simulink model "rlinvpend"  (R2019b)
settings: Solver=VariableStepAuto  StartTime=0.0  StopTime=Tf  RelTol=1e-3
model workspace (MATLAB code in the model file):
  | mCart = 1;
  | mPend = 1;
  | g = 9.81;
  | L = 0.5;
  | theta0 = 180;
  | Kd = 10;
values from neighbouring files (symbols this model uses):
  alpha_a = 0.002    [invertedpndlm_MrAsadmfile.m]
  alpha_c = 0.001    [invertedpndlm_MrAsadmfile.m]
  epsilon = 0.001    [invertedpndlm_MrAsadmfile.m]
  m = 0.1    [invertedpndlm_MrAsadmfile.m]
  s = tf('s')    [invertedpndlm_MrAsadmfile.m]
  Ts = 0.02    [invertedpndlm_MrAsadmfile.m]
undefined symbols (not defined in the file or in its folder): X, Y, Z
libraries: sm_lib x11, nesl_utility x7, fuzblock x3, rllib x2, simulink x2
settings Model: Creator=ndoshi  LastModifiedBy=hp
settings DataIOCC: TimeSaveName=T  SignalLoggingName=LoggedSigs
settings DebuggingCC: ArithmeticOperatorsInVariantConditions=warning
settings SFSimCC: CustomCodeUndefinedFunction=UseInterfaceOnly

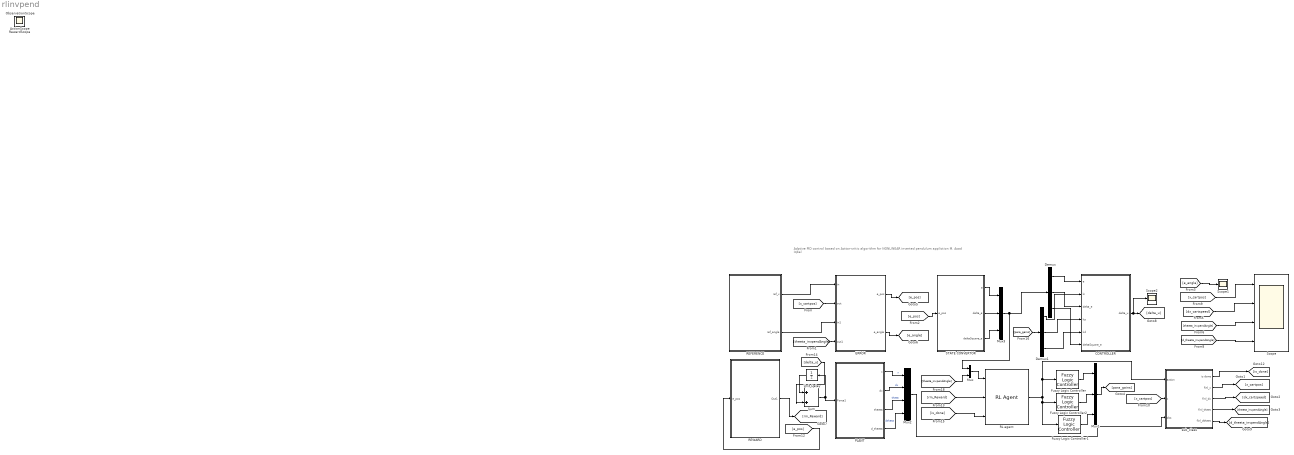
== system rlinvpend ==
  note: Adptive PID control based on Acttor-critic algorithm for NONLINEAR inverted pendulum appliction
      | M. Asad Iqbal
  CONTROLLER : Subsystem
  Demux : Demux  Outputs=3
  Demux1 : Demux  Outputs=3
  ERROR : Subsystem
  Fuzzy Logic Controller : fuzblock/Fuzzy Logic  Controller  FIS=p_n  OutputSampleNumber=101  DataType=double  FuzzifiedInputs=off  RuleFiringStrengths=off  RuleOutputs=off  AggregatedOutputs=off  SimulateUsing=Interpreted execution  OutOfRangeInputValueMessage=warning  NoRuleFiredMessage=warning  EmptyOutputFuzzySetMessage=warning
  Fuzzy Logic Controller1 : fuzblock/Fuzzy Logic  Controller  FIS=d_n  OutputSampleNumber=101  DataType=double  FuzzifiedInputs=off  RuleFiringStrengths=off  RuleOutputs=off  AggregatedOutputs=off  SimulateUsing=Interpreted execution  OutOfRangeInputValueMessage=warning  NoRuleFiredMessage=warning  EmptyOutputFuzzySetMessage=warning
  Fuzzy Logic Controller2 : fuzblock/Fuzzy Logic  Controller  FIS=i_ni  OutputSampleNumber=101  DataType=double  FuzzifiedInputs=off  RuleFiringStrengths=off  RuleOutputs=off  AggregatedOutputs=off  SimulateUsing=Interpreted execution  OutOfRangeInputValueMessage=warning  NoRuleFiredMessage=warning  EmptyOutputFuzzySetMessage=warning
  Mux : Mux  Inputs=2
  Mux1 : Mux  Inputs=3
  Mux2 : Mux
  Mux3 : Mux  Inputs=3
  PLANT : Subsystem
  REFERENCE : Subsystem
  REWARD : Subsystem
  "RL agent " : rllib/RL Agent  Agent=agent  ProvideReward=on  ProvideIsDone=on  ProvideCumRwd=off  TreatAsDirectFeedthrough=on  CollectLoggedSignals=on  CollectModelStates=on
      settings: SourceProductName=The database C:\Users\ddavis\AppData\Roaming\MathWorks\MATLAB\R2018b\slblocks_master.db is locked, or a table in the database is locked. (database is locked)
  STATE CONVERTOR : Subsystem
  Scope : Scope  NumInputPorts=4
  Scope1 : Scope
  Scope2 : Scope
  Sum : Sum  Inputs=|++
  Unit Delay : UnitDelay  SampleTime=-1  HasFrameUpgradeWarning=on
  sub_class : Subsystem
  ActionScope : Scope
  ObservationScope : Scope
  RewardScope : Scope
  wires:
  PLANT/1(x) -> Mux2/1  "x"
  PLANT/4(d_theeta) -> Mux2/4  "dtheta"
  [para_gains] -> Demux1/1
  STATE CONVERTOR/3(deltaSquare_e) -> Mux3/3
  [theeta_invpendAngle] -> ERROR/4(out1)
  Demux/3 -> CONTROLLER/6(deltaSquare_e)
  Demux/1 -> CONTROLLER/1("e ")
  [e_pos] -> REWARD/1(e_pos)
  [d_theeta_invpendAngle] -> Scope/4
  [dx_cartspeed] -> Scope/2
  Demux1/3 -> CONTROLLER/5(kd)
  Unit Delay/1 -> Sum/1
  [theeta_invpendAngle] -> Scope/3
  [x_cartpos] -> Scope/1
  CONTROLLER/1(delta_u) -> Scope2/1, [delta_u]
  Demux1/2 -> CONTROLLER/4(kp)
  Sum/1 -> Unit Delay/1, PLANT/1(Force1)
  [delta_u] -> Sum/2
  Demux/2 -> CONTROLLER/3(delta_e)
  [x_cartpos] -> ERROR/2(out)
  REFERENCE/2(ref_angle) -> ERROR/3(in1)
  STATE CONVERTOR/2(delta_e) -> Mux3/2
  [e_pos] -> STATE CONVERTOR/1("e_pos ")
  ERROR/1(e_pos) -> [e_pos]
  ERROR/2(e_angle) -> [e_angle]
  REFERENCE/1(ref_x) -> ERROR/1(in)
  REWARD/1(Out1) -> [rm_Reward]
  Demux1/1 -> CONTROLLER/2(ki)
  PLANT/2(dx) -> Mux2/2  "dx"
  STATE CONVERTOR/1(e) -> Mux3/1
  PLANT/3(theeta) -> Mux2/3  "theta"
  [theeta_invpendAngle] -> Mux/2
  sub_class/1(is done) -> [is_done]
  sub_class/2(finl_x) -> [x_cartpos]
  sub_class/3(finl_dx) -> [dx_cartspeed]
  Mux/1 -> "RL agent "/1
  [rm_Reward] -> "RL agent "/2
  Mux3/1 -> Mux/1, Demux/1
  [is_done] -> "RL agent "/3
  sub_class/4(finl_theet) -> [theeta_invpendAngle]
  [x_cartpos] -> sub_class/2(x)
  sub_class/5(finl_dtheet) -> [d_theeta_invpendAngle]
  Mux2/1 -> sub_class/3(obs)
  "RL agent "/1 -> sub_class/1("action "), Fuzzy Logic Controller/1, Fuzzy Logic Controller1/1, Fuzzy Logic Controller2/1
  Fuzzy Logic Controller/1 -> Mux1/1
  Fuzzy Logic Controller2/1 -> Mux1/2
  Fuzzy Logic Controller1/1 -> Mux1/3
  [e_angle] -> Scope1/1
  Mux1/1 -> [para_gains]

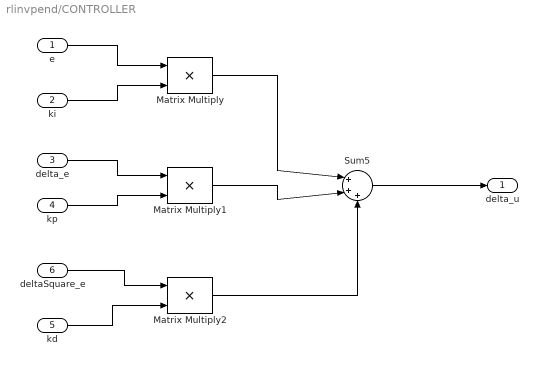
== system rlinvpend/CONTROLLER ==
  "e " : Inport
  ki : Inport  Port=2
  delta_e : Inport  Port=3
  kp : Inport  Port=4
  kd : Inport  Port=5
  deltaSquare_e : Inport  Port=6
  Matrix Multiply : Product
  Matrix Multiply1 : Product
  Matrix Multiply2 : Product
  Sum5 : Sum  Inputs=|+++
  delta_u : Outport
  wires:
  Sum5/1 -> delta_u/1
  deltaSquare_e/1 -> Matrix Multiply2/1
  delta_e/1 -> Matrix Multiply1/1
  "e "/1 -> Matrix Multiply/1
  ki/1 -> Matrix Multiply/2
  kd/1 -> Matrix Multiply2/2
  Matrix Multiply/1 -> Sum5/1
  kp/1 -> Matrix Multiply1/2
  Matrix Multiply1/1 -> Sum5/2
  Matrix Multiply2/1 -> Sum5/3

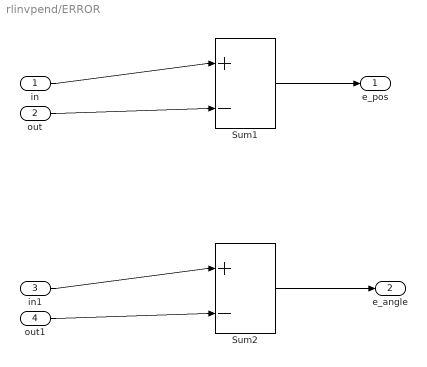
== system rlinvpend/ERROR ==
  in : Inport
  out : Inport  Port=2
  in1 : Inport  Port=3
  out1 : Inport  Port=4
  Sum1 : Sum  Inputs=|+-
  Sum2 : Sum  Inputs=|+-
  e_pos : Outport
  e_angle : Outport  Port=2
  wires:
  in/1 -> Sum1/1
  out/1 -> Sum1/2
  in1/1 -> Sum2/1
  out1/1 -> Sum2/2
  Sum1/1 -> e_pos/1
  Sum2/1 -> e_angle/1

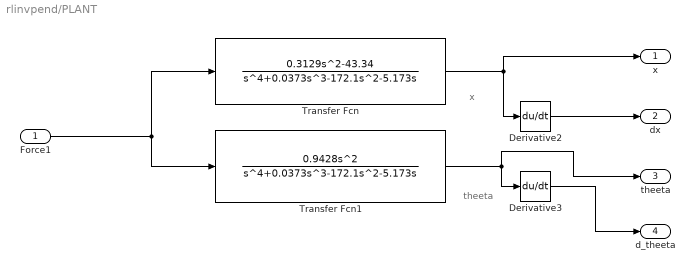
== system rlinvpend/PLANT ==
  note: theeta
  note: x
  Force1 : Inport
  Derivative2 : Derivative
  Derivative3 : Derivative
  Transfer Fcn : TransferFcn  Numerator=[0 0 0.3129 0 -43.34]  Denominator=[1 0.0373 -172.1 -5.173 0]
  Transfer Fcn1 : TransferFcn  Numerator=[0 0 0.9428 0 0]  Denominator=[1 0.0373 -172.1 -5.173 0]
  x : Outport
  dx : Outport  Port=2
  theeta : Outport  Port=3
  d_theeta : Outport  Port=4
  wires:
  Transfer Fcn1/1 -> theeta/1, Derivative3/1
  Transfer Fcn/1 -> x/1, Derivative2/1
  Derivative3/1 -> d_theeta/1
  Derivative2/1 -> dx/1
  Force1/1 -> Transfer Fcn1/1, Transfer Fcn/1

== system rlinvpend/REFERENCE ==
  "Step Input Displacement " : Step  Time=0.005  Before=0.2  After=0  SampleTime=0
  TILT ANGLE : Step  Time=0  After=0  SampleTime=0
  ref_x : Outport
  ref_angle : Outport  Port=2
  wires:
  TILT ANGLE/1 -> ref_angle/1
  "Step Input Displacement "/1 -> ref_x/1

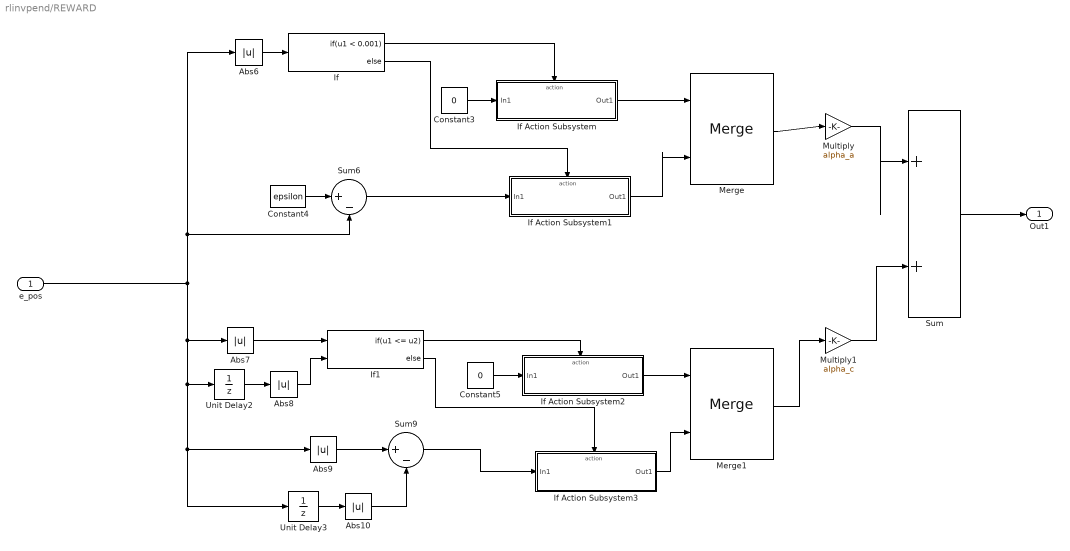
== system rlinvpend/REWARD ==
  e_pos : Inport
  Abs{6..10} (5 alike) : Abs
  Constant3 : Constant  Value=0
  Constant4 : Constant  Value=epsilon
  Constant5 : Constant  Value=0
  If : If  IfExpression=u1 < 0.001
  If Action Subsystem : Subsystem  TreatAsAtomicUnit=on
  If Action Subsystem1 : Subsystem  TreatAsAtomicUnit=on
  If Action Subsystem2 : Subsystem  TreatAsAtomicUnit=on
  If Action Subsystem3 : Subsystem  TreatAsAtomicUnit=on
  If1 : If  NumInputs=2  IfExpression=u1 <= u2
  Merge : Merge
  Merge1 : Merge
  Multiply : Gain  Gain=alpha_a
  Multiply1 : Gain  Gain=alpha_c
  Sum : Sum  Inputs=|++
  Sum6 : Sum  Inputs=|+-
  Sum9 : Sum  Inputs=|+-
  Unit Delay2 : UnitDelay  SampleTime=-1  HasFrameUpgradeWarning=on
  Unit Delay3 : UnitDelay  SampleTime=-1  HasFrameUpgradeWarning=on
  Out1 : Outport
  wires:
  Sum6/1 -> If Action Subsystem1/1(In1)
  If/2 -> If Action Subsystem1/Action
  Constant4/1 -> Sum6/1
  e_pos/1 -> Abs6/1, Sum6/2, Abs9/1, Unit Delay3/1, Unit Delay2/1, Abs7/1
  Unit Delay3/1 -> Abs10/1
  If Action Subsystem/1(Out1) -> Merge/1
  Constant3/1 -> If Action Subsystem/1(In1)
  Multiply1/1 -> Sum/2
  If Action Subsystem3/1(Out1) -> Merge1/2
  Unit Delay2/1 -> Abs8/1
  Sum/1 -> Out1/1
  If/1 -> If Action Subsystem/Action
  If Action Subsystem1/1(Out1) -> Merge/2
  Abs6/1 -> If/1
  Multiply/1 -> Sum/1
  Merge/1 -> Multiply/1
  Merge1/1 -> Multiply1/1
  Sum9/1 -> If Action Subsystem3/1(In1)
  Abs8/1 -> If1/2
  Abs7/1 -> If1/1
  If Action Subsystem2/1(Out1) -> Merge1/1
  Constant5/1 -> If Action Subsystem2/1(In1)
  Abs10/1 -> Sum9/2
  If1/1 -> If Action Subsystem2/Action
  If1/2 -> If Action Subsystem3/Action
  Abs9/1 -> Sum9/1

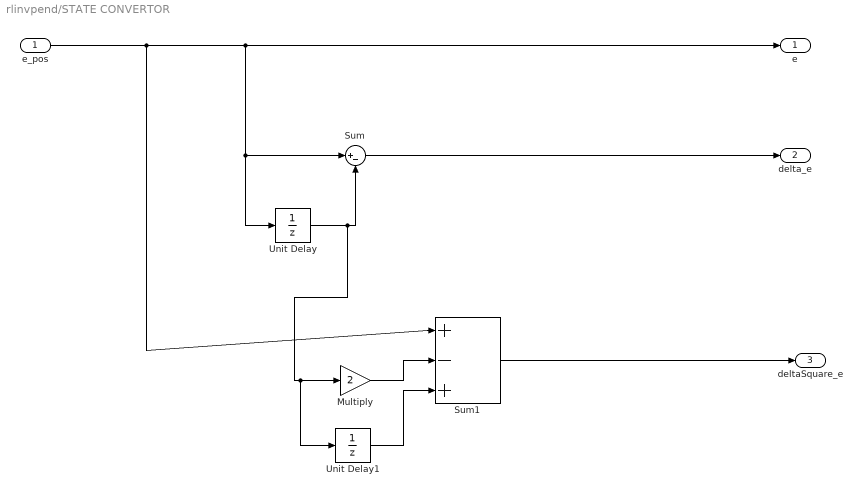
== system rlinvpend/STATE CONVERTOR ==
  "e_pos " : Inport
  Multiply : Gain  Gain=2
  Sum : Sum  Inputs=|+-
  Sum1 : Sum  Inputs=|+-+
  Unit Delay : UnitDelay  SampleTime=-1  HasFrameUpgradeWarning=on
  Unit Delay1 : UnitDelay  SampleTime=-1  HasFrameUpgradeWarning=on
  e : Outport
  delta_e : Outport  Port=2
  deltaSquare_e : Outport  Port=3
  wires:
  "e_pos "/1 -> Sum1/1, Sum/1, Unit Delay/1, e/1
  Unit Delay/1 -> Unit Delay1/1, Multiply/1, Sum/2
  Sum/1 -> delta_e/1
  Sum1/1 -> deltaSquare_e/1
  Multiply/1 -> Sum1/2
  Unit Delay1/1 -> Sum1/3

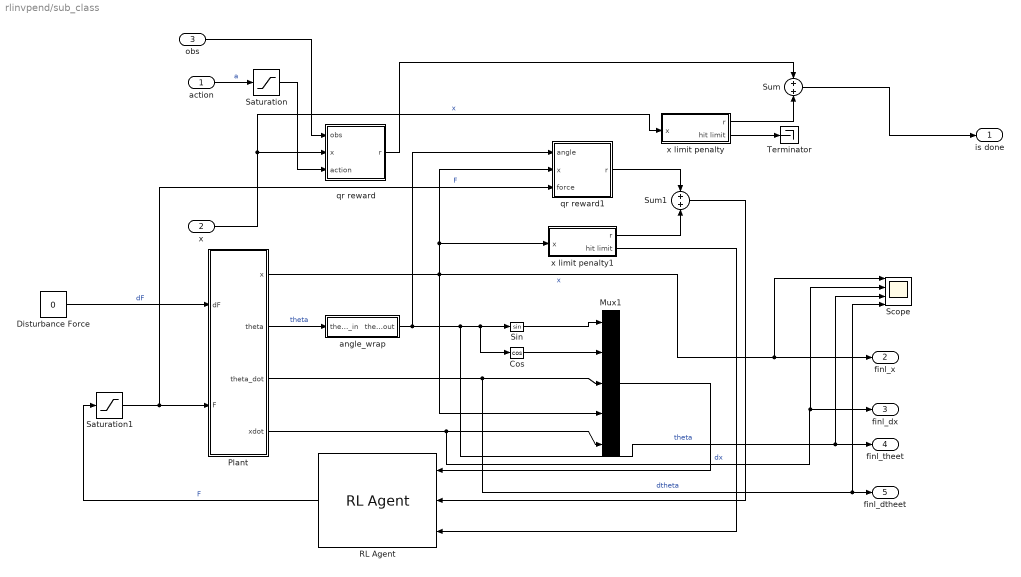
== system rlinvpend/sub_class ==
  "action " : Inport
  x : Inport  Port=2
  obs : Inport  Port=3
  Cos : Trigonometry  Operator=cos
  Disturbance Force : Constant  Value=0
  Mux1 : Mux  Inputs=5
  Plant : Subsystem
  RL Agent : rllib/RL Agent  Agent=agent_dp  ProvideReward=on  ProvideIsDone=on  ProvideCumRwd=off  TreatAsDirectFeedthrough=on  CollectLoggedSignals=on  CollectModelStates=on
      settings: SourceProductName=The database C:\Users\ddavis\AppData\Roaming\MathWorks\MATLAB\R2018b\slblocks_master.db is locked, or a table in the database is locked. (database is locked)
  Saturation : Saturate  UpperLimit=15  LowerLimit=-15
  Saturation1 : Saturate  UpperLimit=15  LowerLimit=-15
  Scope : Scope  NumInputPorts=4
  Sin : Trigonometry
  Sum : Sum
  Sum1 : Sum
  Terminator : Terminator
  angle_wrap : Subsystem
  qr reward : Subsystem
  qr reward1 : Subsystem
  x limit penalty : Subsystem
  x limit penalty1 : Subsystem
  is done : Outport  VectorParamsAs1DForOutWhenUnconnected=off
  finl_x : Outport  Port=2
  finl_dx : Outport  Port=3
  finl_theet : Outport  Port=4
  finl_dtheet : Outport  Port=5
  wires:
  obs/1 -> qr reward/1(obs)
  x/1 -> x limit penalty/1(x), qr reward/2(x)  "x"
  Saturation/1 -> qr reward/3(action)
  "action "/1 -> Saturation/1  "a"
  qr reward/1(r) -> Sum/1
  x limit penalty/1(r) -> Sum/2
  Sum/1 -> is done/1
  x limit penalty1/2(hit limit) -> RL Agent/3
  Sum1/1 -> RL Agent/2
  Mux1/1 -> RL Agent/1
  x limit penalty1/1(r) -> Sum1/2
  qr reward1/1(r) -> Sum1/1
  RL Agent/1 -> Saturation1/1  "F"
  Saturation1/1 -> qr reward1/3(force), Plant/2(F)  "F"
  Cos/1 -> Mux1/2
  Sin/1 -> Mux1/1
  Plant/4(xdot) -> Scope/2, finl_dx/1, Mux1/5  "dx"
  angle_wrap/1(theta_out) -> qr reward1/1(angle), Scope/3, finl_theet/1, Cos/1, Sin/1  "theta"
  Disturbance Force/1 -> Plant/1(dF)  "dF"
  Plant/1(x) -> Scope/1, finl_x/1, Mux1/4, qr reward1/2(x), x limit penalty1/1(x)  "x"
  Plant/2(theta) -> angle_wrap/1(theta_in)  "theta"
  Plant/3(theta_dot) -> Scope/4, finl_dtheet/1, Mux1/3  "dtheta"
  x limit penalty/2(hit limit) -> Terminator/1

== system rlinvpend/REWARD/If Action Subsystem ==
  In1 : Inport
  Action Port : ActionPort  InitializeStates=reset  ActionPortLabel=if(u1 < 0.001)
  Out1 : Outport
  wires:
  In1/1 -> Out1/1

== system rlinvpend/REWARD/If Action Subsystem1 ==
  In1 : Inport
  Action Port : ActionPort  InitializeStates=reset  ActionPortLabel=else
  Out1 : Outport
  wires:
  In1/1 -> Out1/1

== system rlinvpend/REWARD/If Action Subsystem2 ==
  In1 : Inport
  Action Port : ActionPort  InitializeStates=reset  ActionPortLabel=if(u1 <= u2)
  Out1 : Outport
  wires:
  In1/1 -> Out1/1

== system rlinvpend/REWARD/If Action Subsystem3 ==
  In1 : Inport
  Action Port : ActionPort  InitializeStates=reset  ActionPortLabel=else
  Out1 : Outport
  wires:
  In1/1 -> Out1/1

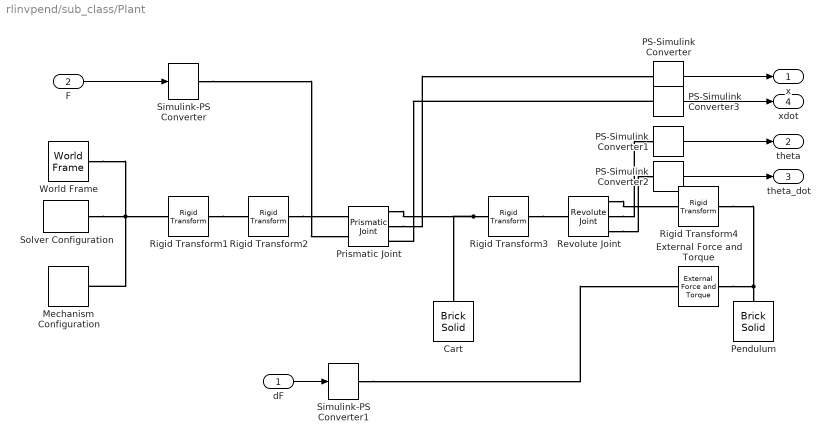
== system rlinvpend/sub_class/Plant ==
  dF : Inport
  F : Inport  Port=2
  Cart : sm_lib/Body Elements/Brick Solid  GraphicAmbientColor=[0.15 0.15 0.15 1.0]  BasedOnType=Density  BrickDimensions=[L/6 L/6 L/3]  BrickDimensionUnits=m  CenterOfMass=[0 0 0]  CenterOfMassUnits=m  GraphicDiffuseColor=[0.5 0.5 0.5]  Density=1000  DensityUnits=kg/(m^3)  DoExposeReferenceFrame=on  GraphicEmissiveColor=[0.0 0.0 0.0 1.0]  ExportEntireGeometry=off  SerializedFrames=<Frames/>  MarkerShape=Sphere  MarkerSize=10  GraphicType=FromGeometry  InertiaType=PointMass  Mass=mCart  MassUnits=kg  MomentsOfInertia=[1 1 1]  MomentsOfInertiaUnits=kg*m^2  GraphicOpacity=1.0  ProductsOfInertia=[0 0 0]  ProductsOfInertiaUnits=kg*m^2  GraphicShininess=75  GraphicSpecularColor=[0.5 0.5 0.5 1.0]  GraphicVisPropType=SimpleVisualProperties
  External Force and Torque : sm_lib/Forces and Torques/External Force and Torque  ForceResolutionFrame=World  EnableForceX=on  EnableForceY=off  EnableForceZ=off  EnableForce=off  TorqueResolutionFrame=AttachedFrame  EnableTorqueX=off  EnableTorqueY=off  EnableTorqueZ=off  EnableTorque=off
  Mechanism Configuration : sm_lib/Utilities/Mechanism Configuration  UniformGravity=Constant  GravityVector=[0 0 -9.81]  GravityUnits=m/s^2  LinearizationDelta=0.001
  PS-Simulink Converter{,1..3} (4 alike) : nesl_utility/PS-Simulink Converter  PhysicalDomain=network_engine_domain  SubClassName=ps_output  LeftPortType=input  RightPortType=output  PseudoPeriodic=off  Frequencies=[]  Unit=1  AffineConversion=off
  Pendulum : sm_lib/Body Elements/Brick Solid  GraphicAmbientColor=[0.15 0.15 0.15 1.0]  BasedOnType=Density  BrickDimensions=[L L/12 L/12]  BrickDimensionUnits=m  CenterOfMass=[0 0 0]  CenterOfMassUnits=m  GraphicDiffuseColor=[0.8 0.0 0.2]  Density=1000  DensityUnits=kg/(m^3)  DoExposeReferenceFrame=on  GraphicEmissiveColor=[0.0 0.0 0.0 1.0]  ExportEntireGeometry=off  SerializedFrames=<Frames/>  MarkerShape=Sphere  MarkerSize=10  GraphicType=FromGeometry  InertiaType=PointMass  Mass=mPend  MassUnits=kg  MomentsOfInertia=[1 1 1]  MomentsOfInertiaUnits=kg*m^2  GraphicOpacity=1.0  ProductsOfInertia=[0 0 0]  ProductsOfInertiaUnits=kg*m^2  GraphicShininess=75  GraphicSpecularColor=[0.5 0.5 0.5 1.0]  GraphicVisPropType=SimpleVisualProperties
  Prismatic Joint : sm_lib/Joints/Prismatic Joint  JointMode=Normal  SenseConstraintForce=off  SenseConstraintForceX=off  SenseConstraintForceY=off  SenseConstraintForceZ=off  SenseConstraintTorque=off  SenseConstraintTorqueX=off  SenseConstraintTorqueY=off  SenseConstraintTorqueZ=off  SenseTotalForce=off  SenseTotalForceX=off  SenseTotalForceY=off  SenseTotalForceZ=off  SenseTotalTorque=off  SenseTotalTorqueX=off  SenseTotalTorqueY=off  SenseTotalTorqueZ=off  CompositeWrenchDir=FollowerOnBase  CompositeWrenchFrame=BaseFrame  EquilibriumPosition=0  EquilibriumPositionUnits=m  SpringStiffness=0  SpringStiffnessUnits=N/m  DampingCoefficient=Kd  DampingCoefficientUnits=N/(m/s)  TorqueActuationMode=InputTorque  MotionActuationMode=ComputedMotion  SensePosition=on  SenseVelocity=on  SenseAcceleration=off  SenseTorqueForce=off  SenseLowerLimitTorqueForce=off  SenseUpperLimitTorqueForce=off  LowerLimitSpecify=off  LowerLimitBound=-1  LowerLimitBoundUnits=m  LowerLimitStiffness=1e6  LowerLimitStiffnessUnits=N/m  LowerLimitDamping=1e3  LowerLimitDampingUnits=N/(m/s)  LowerLimitTransitionRegionWidth=1e-4  LowerLimitTransitionRegionWidthUnits=m  UpperLimitSpecify=off  UpperLimitBound=1  UpperLimitBoundUnits=m  UpperLimitStiffness=1e6  UpperLimitStiffnessUnits=N/m  UpperLimitDamping=1e3  UpperLimitDampingUnits=N/(m/s)  UpperLimitTransitionRegionWidth=1e-4  UpperLimitTransitionRegionWidthUnits=m  PositionTargetSpecify=off  PositionTargetPriority=High  PositionTargetValue=0  PositionTargetValueUnits=m  VelocityTargetSpecify=off  VelocityTargetPriority=High  VelocityTargetValue=0  VelocityTargetValueUnits=m/s
  Revolute Joint : sm_lib/Joints/Revolute Joint  JointMode=Normal  SenseConstraintForce=off  SenseConstraintForceX=off  SenseConstraintForceY=off  SenseConstraintForceZ=off  SenseConstraintTorque=off  SenseConstraintTorqueX=off  SenseConstraintTorqueY=off  SenseConstraintTorqueZ=off  SenseTotalForce=off  SenseTotalForceX=off  SenseTotalForceY=off  SenseTotalForceZ=off  SenseTotalTorque=off  SenseTotalTorqueX=off  SenseTotalTorqueY=off  SenseTotalTorqueZ=off  CompositeWrenchDir=FollowerOnBase  CompositeWrenchFrame=BaseFrame  EquilibriumPosition=0  EquilibriumPositionUnits=deg  SpringStiffness=0  SpringStiffnessUnits=N*m/deg  DampingCoefficient=0  DampingCoefficientUnits=N*m/(rad/s)  TorqueActuationMode=NoTorque  MotionActuationMode=ComputedMotion  SensePosition=on  SenseVelocity=on  SenseAcceleration=off  SenseTorqueForce=off  SenseLowerLimitTorqueForce=off  SenseUpperLimitTorqueForce=off  LowerLimitSpecify=off  LowerLimitBound=-90  LowerLimitBoundUnits=deg  LowerLimitStiffness=1e4  LowerLimitStiffnessUnits=N*m/deg  LowerLimitDamping=10  LowerLimitDampingUnits=N*m/(deg/s)  LowerLimitTransitionRegionWidth=0.1  LowerLimitTransitionRegionWidthUnits=deg  UpperLimitSpecify=off  UpperLimitBound=90  UpperLimitBoundUnits=deg  UpperLimitStiffness=1e4  UpperLimitStiffnessUnits=N*m/deg  UpperLimitDamping=10  UpperLimitDampingUnits=N*m/(deg/s)  UpperLimitTransitionRegionWidth=0.1  UpperLimitTransitionRegionWidthUnits=deg  PositionTargetSpecify=on  PositionTargetPriority=High  PositionTargetValue=theta0  PositionTargetValueUnits=deg  VelocityTargetSpecify=off  VelocityTargetPriority=High  VelocityTargetValue=0  VelocityTargetValueUnits=deg/s
  Rigid Transform1 : sm_lib/Frames and Transforms/Rigid Transform  TranslationMethod=None  TranslationStandardOffset=0  TranslationLengthUnit=m  TranslationStandardAxis=+Z  TranslationCartesianOffset=[0 0 0]  TranslationROffset=0  TranslationROffsetUnits=m  TranslationZOffset=0  TranslationZOffsetUnits=m  TranslationThetaOffset=0  TranslationThetaOffsetUnits=deg  RotationMethod=StandardAxis  RotationAngleUnits=deg  RotationStandardAxis=+Y  RotationAngle=90  RotationArbitraryAxis=[0 0 1]  FollAlignAxisA=+X  BaseAlignAxisA=+Y  FollAlignAxisB=+Y  BaseAlignAxisB=+Z  RotationSequenceAxes=FollowerAxes  RotationSequence=XYX  RotationSequenceAngles=[0 0 0]  RotationSequenceAnglesUnits=deg  RotationMatrix=[1 0 0; 0 1 0; 0 0 1]
  Rigid Transform2 : sm_lib/Frames and Transforms/Rigid Transform  TranslationMethod=None  TranslationStandardOffset=0  TranslationLengthUnit=m  TranslationStandardAxis=+Z  TranslationCartesianOffset=[0 0 0]  TranslationROffset=0  TranslationROffsetUnits=m  TranslationZOffset=0  TranslationZOffsetUnits=m  TranslationThetaOffset=0  TranslationThetaOffsetUnits=deg  RotationMethod=StandardAxis  RotationAngleUnits=deg  RotationStandardAxis=+Z  RotationAngle=180  RotationArbitraryAxis=[0 0 1]  FollAlignAxisA=+X  BaseAlignAxisA=+Y  FollAlignAxisB=+Y  BaseAlignAxisB=+Z  RotationSequenceAxes=FollowerAxes  RotationSequence=XYX  RotationSequenceAngles=[0 0 0]  RotationSequenceAnglesUnits=deg  RotationMatrix=[1 0 0; 0 1 0; 0 0 1]
  Rigid Transform3 : sm_lib/Frames and Transforms/Rigid Transform  TranslationMethod=None  TranslationStandardOffset=0  TranslationLengthUnit=m  TranslationStandardAxis=+Z  TranslationCartesianOffset=[0 0 0]  TranslationROffset=0  TranslationROffsetUnits=m  TranslationZOffset=0  TranslationZOffsetUnits=m  TranslationThetaOffset=0  TranslationThetaOffsetUnits=deg  RotationMethod=StandardAxis  RotationAngleUnits=deg  RotationStandardAxis=-X  RotationAngle=90  RotationArbitraryAxis=[0 0 1]  FollAlignAxisA=+X  BaseAlignAxisA=+Y  FollAlignAxisB=+Y  BaseAlignAxisB=+Z  RotationSequenceAxes=FollowerAxes  RotationSequence=XYX  RotationSequenceAngles=[0 0 0]  RotationSequenceAnglesUnits=deg  RotationMatrix=[1 0 0; 0 1 0; 0 0 1]
  Rigid Transform4 : sm_lib/Frames and Transforms/Rigid Transform  TranslationMethod=StandardAxis  TranslationStandardOffset=L/2  TranslationLengthUnit=m  TranslationStandardAxis=+X  TranslationCartesianOffset=[0 0 0]  TranslationROffset=0  TranslationROffsetUnits=m  TranslationZOffset=0  TranslationZOffsetUnits=m  TranslationThetaOffset=0  TranslationThetaOffsetUnits=deg  RotationMethod=StandardAxis  RotationAngleUnits=deg  RotationStandardAxis=+X  RotationAngle=90  RotationArbitraryAxis=[0 0 1]  FollAlignAxisA=+X  BaseAlignAxisA=+Y  FollAlignAxisB=+Y  BaseAlignAxisB=+Z  RotationSequenceAxes=FollowerAxes  RotationSequence=XYX  RotationSequenceAngles=[0 0 0]  RotationSequenceAnglesUnits=deg  RotationMatrix=[1 0 0; 0 1 0; 0 0 1]
  Simulink-PS Converter : nesl_utility/Simulink-PS Converter  PhysicalDomain=network_engine_domain  SubClassName=ps_input  LeftPortType=input  RightPortType=output  PseudoPeriodic=off  Frequencies=[]  NoiseDistribution=none  NoiseParameters=[]  Unit=1  AffineConversion=off  FilteringAndDerivatives=zero  SimscapeFilterOrder=1  InputFilterTimeConstant=0.001  UdotUserProvided=1
  Simulink-PS Converter1 : nesl_utility/Simulink-PS Converter  PhysicalDomain=network_engine_domain  SubClassName=ps_input  LeftPortType=input  RightPortType=output  PseudoPeriodic=off  Frequencies=[]  NoiseDistribution=none  NoiseParameters=[]  Unit=1  AffineConversion=off  FilteringAndDerivatives=zero  SimscapeFilterOrder=1  InputFilterTimeConstant=0.001  UdotUserProvided=1
  Solver Configuration : nesl_utility/Solver Configuration  PhysicalDomain=network_engine_domain  SubClassName=solver  LeftPortType=input  RightPortType=generic  Tones=[]  Harmonics=[]  SimulateNoise=off  Profile=off  UseLocalSampling=off  EnableSwitchedLinearOptims=on  FrequencyDomain=off  UseCCode=off  RelTol=0.001  AbsTol=1e-06  MinStep=1e-09  ToWorkspace=off  RevertToSquareIcSolve=off  NumHomotopyIterations=100  PhasorMode=off  PhasorModeNumHarmonics=1  DoDC=off  ResidualTolerance=1e-09  UseLocalSolver=off  LocalSolverChoice=NE_BACKWARD_EULER_ADVANCER  LocalSolverSampleTime=0.001  DoFixedCost=off  MaxNonlinIter=3  MaxModeIter=2  LinearAlgebra=Sparse  EquationFormulation=NE_TIME_EF  DelaysMemoryBudget=1024  AutomaticFiltering=on  FilteringTimeConstant=0.001  PartitionStorageMethod=AS_NEEDED  PartitionMemoryBudget=1024  PartitionMethod=FAST
  World Frame : sm_lib/Frames and Transforms/World Frame
  x : Outport  VectorParamsAs1DForOutWhenUnconnected=off
  theta : Outport  Port=2  VectorParamsAs1DForOutWhenUnconnected=off
  theta_dot : Outport  Port=3  VectorParamsAs1DForOutWhenUnconnected=off
  xdot : Outport  Port=4  VectorParamsAs1DForOutWhenUnconnected=off
  wires:
  PS-Simulink Converter1/1 -> theta/1
  PS-Simulink Converter/1 -> x/1
  F/1 -> Simulink-PS Converter/1
  dF/1 -> Simulink-PS Converter1/1
  PS-Simulink Converter2/1 -> theta_dot/1
  PS-Simulink Converter3/1 -> xdot/1
  connections:
  Rigid Transform3/LConn1 -- Cart/RConn1 -- Prismatic Joint/RConn1
  World Frame/RConn1 -- Solver Configuration/RConn1 -- Mechanism Configuration/RConn1 -- Rigid Transform1/LConn1
  Revolute Joint/RConn1 -- Rigid Transform4/LConn1
  Rigid Transform4/RConn1 -- External Force and Torque/RConn1 -- Pendulum/RConn1
  Rigid Transform3/RConn1 -- Revolute Joint/LConn1
  Revolute Joint/RConn2 -- PS-Simulink Converter1/LConn1
  Prismatic Joint/RConn2 -- PS-Simulink Converter/LConn1
  Simulink-PS Converter/RConn1 -- Prismatic Joint/LConn2
  Simulink-PS Converter1/RConn1 -- External Force and Torque/LConn1
  Rigid Transform1/RConn1 -- Rigid Transform2/LConn1
  Rigid Transform2/RConn1 -- Prismatic Joint/LConn1
  Revolute Joint/RConn3 -- PS-Simulink Converter2/LConn1
  PS-Simulink Converter3/LConn1 -- Prismatic Joint/RConn3

== system rlinvpend/sub_class/angle_wrap ==
  theta_in : Inport
  Trigonometric Function : Trigonometry  Operator=atan2
  Trigonometric Function1 : Trigonometry
  Trigonometric Function2 : Trigonometry  Operator=cos
  theta_out : Outport  VectorParamsAs1DForOutWhenUnconnected=off
  wires:
  theta_in/1 -> Trigonometric Function2/1, Trigonometric Function1/1
  Trigonometric Function/1 -> theta_out/1
  Trigonometric Function1/1 -> Trigonometric Function/1
  Trigonometric Function2/1 -> Trigonometric Function/2

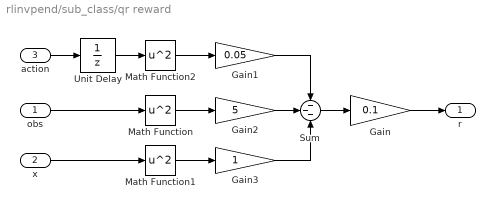
== system rlinvpend/sub_class/qr reward ==
  obs : Inport
  x : Inport  Port=2
  action : Inport  Port=3
  Gain : Gain  Gain=0.1
  Gain1 : Gain  Gain=0.05
  Gain2 : Gain  Gain=5
  Gain3 : Gain
  Math Function : Math  Operator=square  SaturateOnIntegerOverflow=on
  Math Function1 : Math  Operator=square  SaturateOnIntegerOverflow=on
  Math Function2 : Math  Operator=square  SaturateOnIntegerOverflow=on
  Sum : Sum  Inputs=---
  Unit Delay : UnitDelay  SampleTime=0.0002  HasFrameUpgradeWarning=on
  r : Outport  VectorParamsAs1DForOutWhenUnconnected=off
  wires:
  obs/1 -> Math Function/1
  Gain2/1 -> Sum/2
  Gain3/1 -> Sum/3
  Math Function2/1 -> Gain1/1
  Math Function1/1 -> Gain3/1
  action/1 -> Unit Delay/1
  x/1 -> Math Function1/1
  Math Function/1 -> Gain2/1
  Gain1/1 -> Sum/1
  Sum/1 -> Gain/1
  Unit Delay/1 -> Math Function2/1
  Gain/1 -> r/1

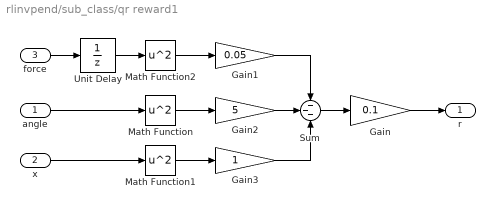
== system rlinvpend/sub_class/qr reward1 ==
  angle : Inport
  x : Inport  Port=2
  force : Inport  Port=3
  Gain : Gain  Gain=0.1
  Gain1 : Gain  Gain=0.05
  Gain2 : Gain  Gain=5
  Gain3 : Gain
  Math Function : Math  Operator=square  SaturateOnIntegerOverflow=on
  Math Function1 : Math  Operator=square  SaturateOnIntegerOverflow=on
  Math Function2 : Math  Operator=square  SaturateOnIntegerOverflow=on
  Sum : Sum  Inputs=---
  Unit Delay : UnitDelay  SampleTime=Ts  HasFrameUpgradeWarning=on
  r : Outport  VectorParamsAs1DForOutWhenUnconnected=off
  wires:
  angle/1 -> Math Function/1
  Gain2/1 -> Sum/2
  Gain3/1 -> Sum/3
  Math Function2/1 -> Gain1/1
  Math Function1/1 -> Gain3/1
  force/1 -> Unit Delay/1
  x/1 -> Math Function1/1
  Math Function/1 -> Gain2/1
  Gain1/1 -> Sum/1
  Sum/1 -> Gain/1
  Unit Delay/1 -> Math Function2/1
  Gain/1 -> r/1

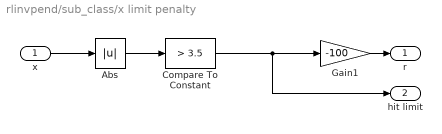
== system rlinvpend/sub_class/x limit penalty ==
  x : Inport
  Abs : Abs
  Compare To Constant : simulink/Logic and Bit Operations/Compare To Constant  relop=>  const=3.5  OutDataTypeStr=boolean
  Gain1 : Gain  Gain=-100
  r : Outport  VectorParamsAs1DForOutWhenUnconnected=off
  hit limit : Outport  Port=2  VectorParamsAs1DForOutWhenUnconnected=off
  wires:
  Gain1/1 -> r/1
  x/1 -> Abs/1
  Abs/1 -> Compare To Constant/1
  Compare To Constant/1 -> hit limit/1, Gain1/1

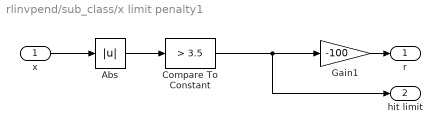
== system rlinvpend/sub_class/x limit penalty1 ==
  x : Inport
  Abs : Abs
  Compare To Constant : simulink/Logic and Bit Operations/Compare To Constant  relop=>  const=3.5  OutDataTypeStr=boolean
  Gain1 : Gain  Gain=-100
  r : Outport  VectorParamsAs1DForOutWhenUnconnected=off
  hit limit : Outport  Port=2  VectorParamsAs1DForOutWhenUnconnected=off
  wires:
  Gain1/1 -> r/1
  x/1 -> Abs/1
  Abs/1 -> Compare To Constant/1
  Compare To Constant/1 -> hit limit/1, Gain1/1
